simulink model "sl_subsys_fcncall3"  (Simulink 6.0)
settings: Solver=FixedStepDiscrete  StartTime=0.0  StopTime=10.0  FixedStep=1  RelTol=1e-3
settings Model: CovMetricSettings=d  Creator=The MathWorks Inc.  LastModifiedBy=batserve  ExtModeAutoUpdateStatusClock=off
settings DataIOCC: SignalLoggingName=logsOut
settings OptimizationCC: BlockReduction=off  BooleanDataType=off
settings DebuggingCC: CheckExecutionContextPreStartOutputMsg=on  CheckExecutionContextRuntimeOutputMsg=on  SolverPrmCheckMsg=none
settings HardwareCC: TargetUnknown=on

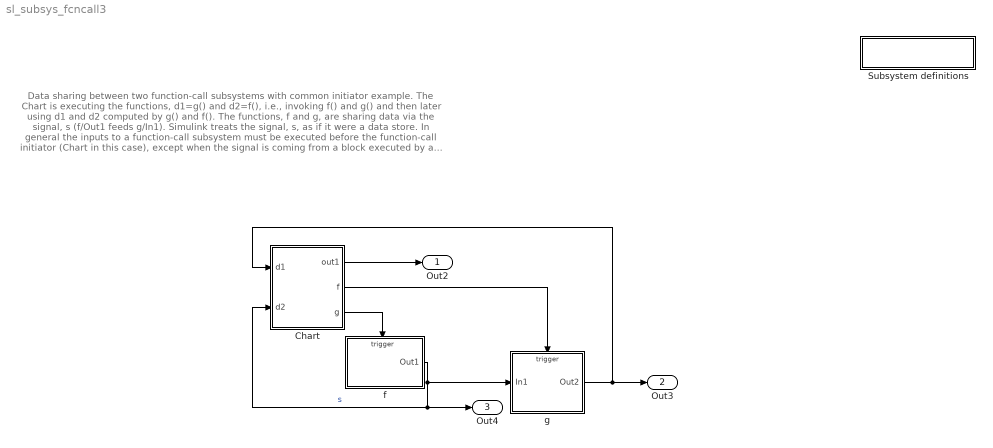
== system sl_subsys_fcncall3 ==
  note: Data sharing between two function-call subsystems with common initiator example.
      |
      | The Chart is executing the functions, d1=g() and d2=f(), i.e., invoking
      | f() and g() and then later using d1 and d2 computed by g() and f().
      | The functions, f and g, are sharing data via the signal, s (f/Out1 feeds g/In1).
      | Simulink treats the signal, s, as if it were a data store.
      |
      | In general the inputs to a function-call subsystem must be executed before the
      | function-call initiator (Chart in this case), except when the signal is coming
      | from a block executed by a common function-call initiator. For our example,
      | Chart is a common function-call initiator of both f() and g(). Therefore,
      | the signal, s, below can be thought of as a data store.
  " Subsystem definitions" : Subsystem  PropExecContextAcrossSSBoundary=on
      settings: OpenFcn=helpview([matlabroot,'/toolbox/simulink/simdemos/sl_subsys_definitions.html']);
      mask Display: disp('Subsystem\ndefinitions')
  Chart : Stateflow chart  PropExecContextAcrossSSBoundary=on
  f : Subsystem  TreatAsAtomicUnit=on  PropExecContextAcrossSSBoundary=on
  g : Subsystem  TreatAsAtomicUnit=on  PropExecContextAcrossSSBoundary=on
  Out2 : Outport
  Out3 : Outport  Port=2
  Out4 : Outport  Port=3
  wires:
  Chart/3(g) -> f/Trigger
  f/1(Out1) -> g/1(In1), Out4/1, Chart/2(d2)  "s"
  g/1(Out2) -> Out3/1, Chart/1(d1)
  Chart/1(out1) -> Out2/1
  Chart/2(f) -> g/Trigger

== system sl_subsys_fcncall3/ Subsystem definitions ==

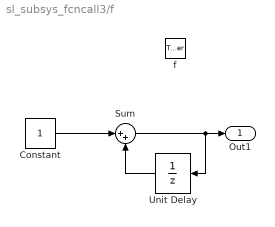
== system sl_subsys_fcncall3/f ==
  f : TriggerPort  TriggerType=function-call  StatesWhenEnabling=reset
  Constant : Constant
  Sum : Sum  Inputs=|++  SaturateOnIntegerOverflow=on  InputSameDT=on
  Unit Delay : UnitDelay  Orientation=left  SampleTime=-1
  Out1 : Outport
  wires:
  Constant/1 -> Sum/1
  Unit Delay/1 -> Sum/2
  Sum/1 -> Out1/1, Unit Delay/1

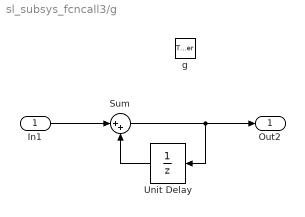
== system sl_subsys_fcncall3/g ==
  In1 : Inport  Port=1  LatchInput=off
  g : TriggerPort  TriggerType=function-call  StatesWhenEnabling=reset
  Sum : Sum  Inputs=|++  SaturateOnIntegerOverflow=on  InputSameDT=on
  Unit Delay : UnitDelay  Orientation=left  SampleTime=-1
  Out2 : Outport
  wires:
  In1/1 -> Sum/1
  Unit Delay/1 -> Sum/2
  Sum/1 -> Out2/1, Unit Delay/1

== stateflow chart Chart ==
  state one/
    entry: f; out1= d1+d2;
  state two/
    entry: g; out1=d1-d2;
  one -> two
  two -> one
  (default) -> one
  data: d1 input double; d2 input double; out1 output double
  events: f output FUNCTION_CALL_EVENT; g output FUNCTION_CALL_EVENT
